simulink model "katayamacopter"  (R2022a)
settings: Solver=VariableStepAuto  StartTime=0.0  StopTime=50  RelTol=1e-3
values from neighbouring files (symbols this model uses):
  A_elev = [0  1; 0  -0.11]    [param.mat]
  A_pitch = [0  1; 0  0]    [param.mat]
  A_travel = [0  1; 0  -0.0247]    [param.mat]
  B_elev = [0  0; 0.655  0]    [param.mat]
  B_pitch = [0  0; 0  0.248]    [param.mat]
  B_travel = [0  0; 0.0086  0]    [param.mat]
  C_elev = [1  0; 0  0]    [param.mat]
  C_pitch = [1  0; 0  0]    [param.mat]
  C_travel = [1  0; 0  0]    [param.mat]
  D_elev = [0  0; 0  0]    [param.mat]
  D_pitch = [0  0; 0  0]    [param.mat]
  D_travel = [0  0; 0  0]    [param.mat]
undefined symbols (not defined in the file or in its folder): pitch_min
libraries: mpclib x3
settings Model: VariantFading=off  Creator=marik  LastModifiedBy=marik
settings DebuggingCC: UnderSpecifiedDimensionMsg=warning

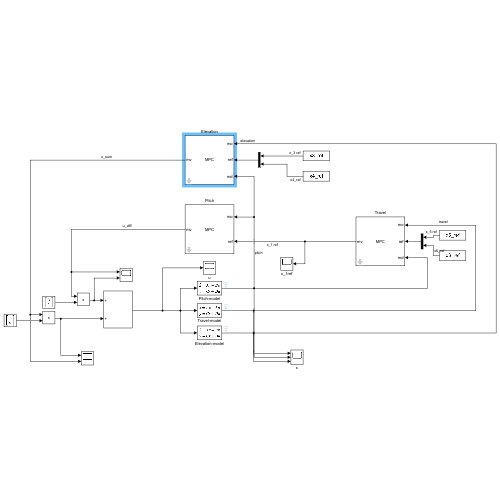
[thumbnail: Simulink's stored preview of the top-level diagram]
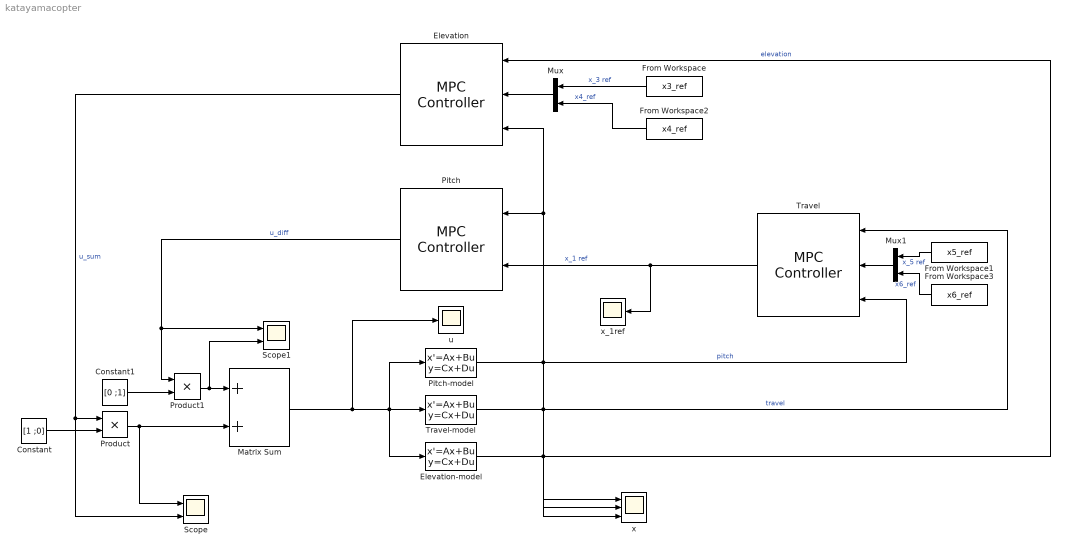
== system katayamacopter ==
  Constant : Constant  Value=[1 ;0]  VectorParams1D=off
  Constant1 : Constant  Value="[0  ;1]"  VectorParams1D=off
  Elevation : mpclib/MPC Controller  SCDEnableBlockLinearizationSpecification=on  mpcobj=mpcelev  is_multiple=0  enable_value=0  return_u0=off  updateMPCinCallerWorkspace=on  md_inport=on  mv_inport=off  uref_inport=off  return_cost=off  return_mvseq=off  return_qpstatus=off  return_xseq=off  return_state=off  return_ovseq=off  state_inport=off  umin_inport=off  umax_inport=off  ymin_inport=off  ymax_inport=off  cc_inport=off  ywt_inport=off  uwt_inport=off  duwt_inport=off  rhoeps_inport=off  pm_inport=off  MaximumP=10  HorizonChoice=FixedHorizon  n_ts=0.02  n_p=30  n_mv=2  n_md=1  n_ud=0  n_mo=2  n_uo=0  BlockDataType=double  SampleTimeInherited=off  switch_inport=off
  Elevation-model : StateSpace  A=A_elev  B=B_elev  C=C_elev  D=D_elev  InitialCondition=pitch_min
  From Workspace : FromWorkspace  VariableName=x3_ref  SampleTime=0.1  OutputAfterFinalValue=Holding final value
  From Workspace1 : FromWorkspace  VariableName=x5_ref  SampleTime=0.1  OutputAfterFinalValue=Holding final value
  From Workspace2 : FromWorkspace  VariableName=x4_ref
  From Workspace3 : FromWorkspace  VariableName=x6_ref
  Matrix Sum : Sum
  Mux : Mux  Inputs=2
  Mux1 : Mux  Inputs=2
  Pitch : mpclib/MPC Controller  SCDEnableBlockLinearizationSpecification=on  mpcobj=mpcpitch  is_multiple=0  enable_value=0  return_u0=off  updateMPCinCallerWorkspace=on  md_inport=off  mv_inport=off  uref_inport=off  return_cost=off  return_mvseq=off  return_qpstatus=off  return_xseq=off  return_state=off  return_ovseq=off  state_inport=off  umin_inport=off  umax_inport=off  ymin_inport=off  ymax_inport=off  cc_inport=off  ywt_inport=off  uwt_inport=off  duwt_inport=off  rhoeps_inport=off  pm_inport=off  MaximumP=10  HorizonChoice=FixedHorizon  n_ts=0.008  n_p=80  n_mv=2  n_md=0  n_ud=0  n_mo=2  n_uo=0  BlockDataType=double  SampleTimeInherited=off  switch_inport=off
  Pitch-model : StateSpace  A=A_pitch  B=B_pitch  C=C_pitch  D=D_pitch  InitialCondition=0
  Product : Product
  Product1 : Product
  Scope : Scope  NumInputPorts=2
  Scope1 : Scope  NumInputPorts=2
  Travel : mpclib/MPC Controller  SCDEnableBlockLinearizationSpecification=on  mpcobj=mpctravel  is_multiple=0  enable_value=0  return_u0=off  updateMPCinCallerWorkspace=on  md_inport=on  mv_inport=off  uref_inport=off  return_cost=off  return_mvseq=off  return_qpstatus=off  return_xseq=off  return_state=off  return_ovseq=off  state_inport=off  umin_inport=off  umax_inport=off  ymin_inport=off  ymax_inport=off  cc_inport=off  ywt_inport=off  uwt_inport=off  duwt_inport=off  rhoeps_inport=off  pm_inport=off  MaximumP=10  HorizonChoice=FixedHorizon  n_ts=0.008  n_p=80  n_mv=2  n_md=1  n_ud=0  n_mo=2  n_uo=0  BlockDataType=double  SampleTimeInherited=off  switch_inport=off
  Travel-model : StateSpace  A=A_travel  B=B_travel  C=C_travel  D=D_travel  InitialCondition=0
  u : Scope
  x : Scope  NumInputPorts=3
  x_1ref : Scope
  wires:
  Travel/1 -> x_1ref/1, Pitch/2  "x_1 ref"
  From Workspace/1 -> Mux/1  "x_3 ref"
  Elevation-model/1 -> x/1, Elevation/1  "elevation"
  Pitch-model/1 -> x/2, Travel/3, Elevation/3, Pitch/1  "pitch"
  Travel-model/1 -> x/3, Travel/1  "travel"
  From Workspace1/1 -> Mux1/1  "x_5 ref"
  Elevation/1 -> Scope/2, Product/1  "u_sum"
  Pitch/1 -> Product1/1, Scope1/1  "u_diff"
  Matrix Sum/1 -> u/1, Pitch-model/1, Travel-model/1, Elevation-model/1
  From Workspace2/1 -> Mux/2  "x4_ref"
  Mux/1 -> Elevation/2
  Mux1/1 -> Travel/2
  From Workspace3/1 -> Mux1/2  "x6_ref"
  Constant/1 -> Product/2
  Product/1 -> Scope/1, Matrix Sum/2
  Constant1/1 -> Product1/2
  Product1/1 -> Scope1/2, Matrix Sum/1
